simulink model "px4demo_gps"  (R2014b)
settings: Solver=ode3  SolverMode=SingleTasking  StartTime=0.0  StopTime=inf  FixedStep=1/250  RelTol=1e-3
PostLoadFcn:
  | Ts = 1/250;
undefined symbols (not defined in the file): RGBLED_COLOR_ENUM, RGBLED_MODE_ENUM
libraries: pixhawk_sllib x2
settings Model: Creator=skuznick  LastModifiedBy=skuznick
settings OptimizationCC: InlineParams=on  OptimizeModelRefInitCode=on  LifeSpan=1  MaxStackSize=64
settings HardwareCC: ProdLargestAtomicInteger=Long  ProdLargestAtomicFloat=Double  ProdEndianess=LittleEndian  ProdLongLongMode=on  ProdHWDeviceType=ARM Compatible->ARM Cortex
settings RTWCC: SystemTargetFile=ert.tlc  TLCOptions=-aInlineSetEventsForThisBaseRateFcn=TLC_FALSE -aSuppressMultiTaskScheduler=TLC_FALSE  TemplateMakefile=ert_default_tmf  Description=Embedded Coder  GenerateReport=on  ProcessScript=ert_make_rtw_hook  Toolchain=Pixhawk Toolchain  IncludeHyperlinkInReport=on  LaunchReport=on  GenerateTraceReport=on  GenerateCodeMetricsReport=on
settings CodeAppCC: IgnoreCustomStorageClasses=off

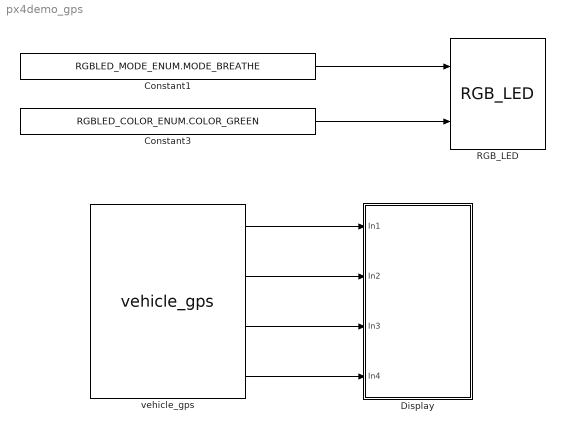
== system px4demo_gps ==
  Constant1 : Constant  Value=RGBLED_MODE_ENUM.MODE_BREATHE  OutDataTypeStr=Enum: RGBLED_MODE_ENUM
  Constant3 : Constant  Value=RGBLED_COLOR_ENUM.COLOR_GREEN  OutDataTypeStr=Enum: RGBLED_COLOR_ENUM
  Display : Subsystem  TreatAsAtomicUnit=on  SystemSampleTime=1
  RGB_LED : pixhawk_sllib/RGB_LED
  vehicle_gps : pixhawk_sllib/vehicle_gps  sampletime=1/250  show_ts_pos=on  show_alt=on  show_ts_gps=off  show_vel=off  show_fixtype=off  show_numsat=off
  wires:
  vehicle_gps/1 -> Display/1(In1)
  vehicle_gps/2 -> Display/2(In2)
  vehicle_gps/3 -> Display/3(In3)
  vehicle_gps/4 -> Display/4(In4)
  Constant1/1 -> RGB_LED/1
  Constant3/1 -> RGB_LED/2

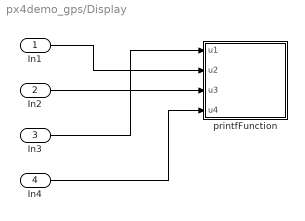
== system px4demo_gps/Display ==
  In1 : Inport
  In2 : Inport  Port=2
  In3 : Inport  Port=3
  In4 : Inport  Port=4
  printfFunction : MATLAB Function  TreatAsAtomicUnit=on
  wires:
  In3/1 -> printfFunction/1(u1)
  In1/1 -> printfFunction/2(u2)
  In4/1 -> printfFunction/4(u4)
  In2/1 -> printfFunction/3(u3)

== matlab function px4demo_gps/Display/printfFunction ==
  data: u1 input double; u2 input int32; u3 input int32; u4 input int32
function fcn(u1, u2, u3, u4)
%#codegen

if strcmp(coder.target, 'rtw') == true
    coder.ceval('printf','GPS->TS: %lld LatLon:[%d %d] Alt:%d %c%c', uint64(u1), u2, u3, u4, uint8(13), uint8(10));
end
